simulink model "Test_Linear_system"  (R2022b)
settings: Solver=VariableStepAuto  StartTime=0.0  StopTime=50  RelTol=1e-3
values from neighbouring files (symbols this model uses):
  A = double(A)    [sys_Modelling.m]
  B = double(B)    [sys_Modelling.m]
  C = zeros((N+1)*n, N*p)    [MPC_Matrices.m]    (also in sys_Modelling.m = double(C))
  D = double(D)    [sys_Modelling.m]
  L = place(sys.A', sys.C',ew_L)'    [Controller_Observer.m]    (also in LQR_Luenberger.m)
  V = -pinv(sys.C*inv(sys.A - sys.B*K)*sys.B)    [Controller_Observer.m]    (also in LQR_Luenberger.m)
undefined symbols (not defined in the file or in its folder): K_neu, u_ap
libraries: simulink_extras x2
settings Model: Creator=renzhijian  LastModifiedBy=12056

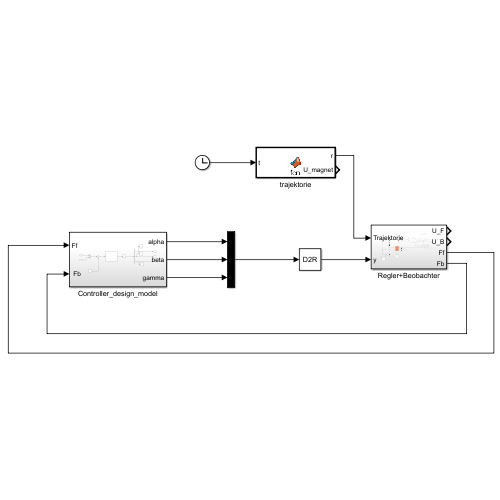
[thumbnail: Simulink's stored preview of the top-level diagram]
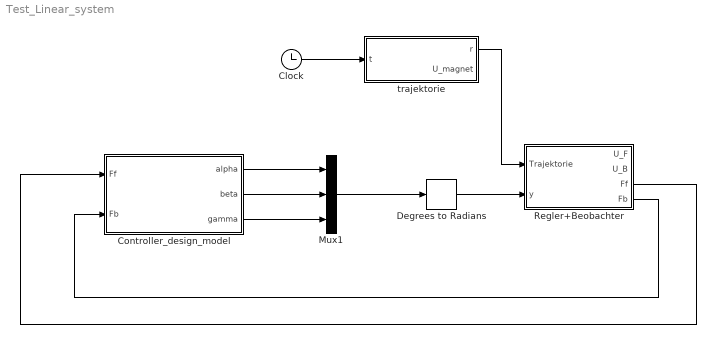
== system Test_Linear_system ==
  Clock : Clock
  Controller_design_model : Subsystem
  Degrees to Radians : simulink_extras/Transformations/Degrees to Radians
  Mux1 : Mux  Inputs=3
  Regler+Beobachter : Subsystem
  trajektorie : MATLAB Function  TreatAsAtomicUnit=on
  wires:
  Controller_design_model/1(alpha) -> Mux1/1
  trajektorie/1(r) -> Regler+Beobachter/1(Trajektorie)
  Regler+Beobachter/3(Ff) -> Controller_design_model/1(Ff)
  Controller_design_model/2(beta) -> Mux1/2
  Controller_design_model/3(gamma) -> Mux1/3
  Regler+Beobachter/4(Fb) -> Controller_design_model/2(" Fb")
  Clock/1 -> trajektorie/1(t)
  Mux1/1 -> Degrees to Radians/1
  Degrees to Radians/1 -> Regler+Beobachter/2(y)

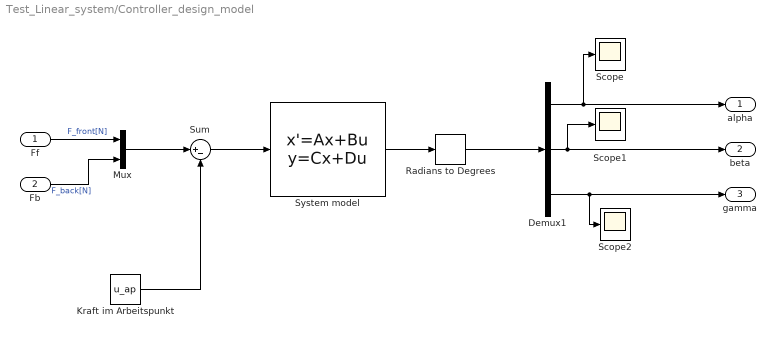
== system Test_Linear_system/Controller_design_model ==
  Ff : Inport
  " Fb" : Inport  Port=2
  Demux1 : Demux  Outputs=3
  Kraft im Arbeitspunkt : Constant  Value=u_ap
  Mux : Mux  Inputs=2
  Radians to Degrees : simulink_extras/Transformations/Radians to Degrees
  Scope : Scope
  Scope1 : Scope
  Scope2 : Scope
  Sum : Sum  Inputs=|+-
  System model : StateSpace  A=A  B=B  C=C  D=D  InitialCondition=[0;-27*pi/180;0;0;0;0]
  alpha : Outport  VectorParamsAs1DForOutWhenUnconnected=off
  beta : Outport  Port=2  VectorParamsAs1DForOutWhenUnconnected=off
  gamma : Outport  Port=3  VectorParamsAs1DForOutWhenUnconnected=off
  wires:
  " Fb"/1 -> Mux/2  "F_back[N]"
  Kraft im Arbeitspunkt/1 -> Sum/2
  System model/1 -> Radians to Degrees/1
  Sum/1 -> System model/1
  Mux/1 -> Sum/1
  Demux1/2 -> beta/1, Scope1/1
  Demux1/3 -> Scope2/1, gamma/1
  Ff/1 -> Mux/1  "F_front[N]"
  Demux1/1 -> Scope/1, alpha/1
  Radians to Degrees/1 -> Demux1/1

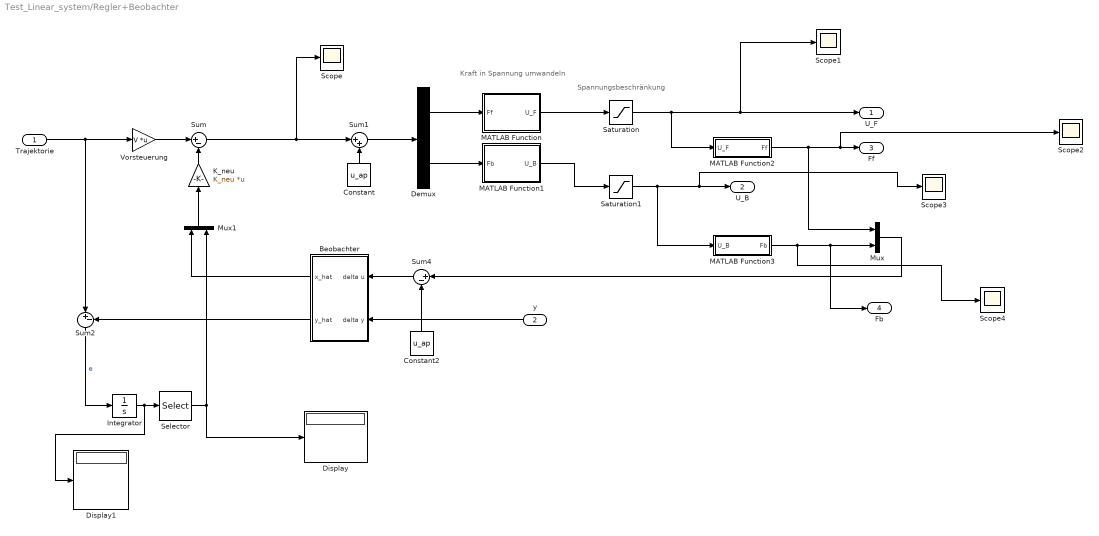
== system Test_Linear_system/Regler+Beobachter ==
  note: Spannungsbeschränkung
  note: Kraft in Spannung umwandeln
  Trajektorie : Inport
  y : Inport  Port=2
  Beobachter : Subsystem
  Constant : Constant  Value=u_ap
  Constant2 : Constant  Value=u_ap
  Demux : Demux  Outputs=2
  Display : Display
  Display1 : Display
  Integrator : Integrator
  K_neu : Gain  Gain=K_neu  Multiplication=Matrix(K*u) (u vector)
  MATLAB Function : MATLAB Function  TreatAsAtomicUnit=on
  MATLAB Function1 : MATLAB Function  TreatAsAtomicUnit=on
  MATLAB Function2 : MATLAB Function  TreatAsAtomicUnit=on
  MATLAB Function3 : MATLAB Function  TreatAsAtomicUnit=on
  Mux : Mux  Inputs=2
  Mux1 : Mux  Inputs=2
  Saturation : Saturate  UpperLimit=4  LowerLimit=0
  Saturation1 : Saturate  UpperLimit=4  LowerLimit=0
  Scope{,1..4} (5 alike) : Scope
  Selector : Selector  InputPortWidth=3  IndexOptions=Index vector (dialog)  Indices=[1 2]  OutputSizes=1
  Sum : Sum  Inputs=|+-
  Sum1 : Sum  Inputs=|++
  Sum2 : Sum  Inputs=|+-
  Sum4 : Sum  Inputs=|+-
  Vorsteuerung : Gain  Gain=V  Multiplication=Matrix(K*u) (u vector)
  U_F : Outport
  U_B : Outport  Port=2
  Ff : Outport  Port=3
  Fb : Outport  Port=4
  wires:
  MATLAB Function1/1(U_B) -> Saturation1/1
  y/1 -> Beobachter/2(delta y)
  Saturation1/1 -> MATLAB Function3/1(U_B), Scope3/1, U_B/1
  Demux/1 -> MATLAB Function/1(Ff)
  Sum1/1 -> Demux/1
  Saturation/1 -> Scope1/1, U_F/1, MATLAB Function2/1(U_F)
  Mux/1 -> Sum4/1
  MATLAB Function2/1(Ff) -> Scope2/1, Ff/1, Mux/1
  MATLAB Function3/1(Fb) -> Scope4/1, Fb/1, Mux/2
  Constant2/1 -> Sum4/2
  Constant/1 -> Sum1/2
  MATLAB Function/1(U_F) -> Saturation/1
  Sum4/1 -> Beobachter/1(delta u)
  Demux/2 -> MATLAB Function1/1(Fb)
  Trajektorie/1 -> Vorsteuerung/1, Sum2/1
  Sum/1 -> Scope/1, Sum1/1
  Sum2/1 -> Integrator/1  "e"
  Integrator/1 -> Display1/1, Selector/1
  Beobachter/2(y_hat) -> Sum2/2
  Beobachter/1(x_hat) -> Mux1/1
  Mux1/1 -> K_neu/1
  K_neu/1 -> Sum/2
  Vorsteuerung/1 -> Sum/1
  Selector/1 -> Mux1/2, Display/1

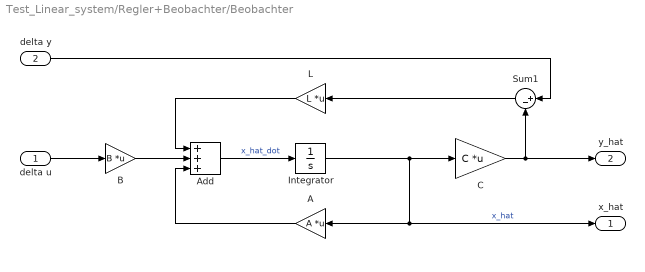
== system Test_Linear_system/Regler+Beobachter/Beobachter ==
  delta u : Inport
  delta y : Inport  Port=2
  A : Gain  Gain=A  Multiplication=Matrix(K*u) (u vector)
  Add : Sum  Inputs=+++
  B : Gain  Gain=B  Multiplication=Matrix(K*u) (u vector)
  C : Gain  Gain=C  Multiplication=Matrix(K*u) (u vector)
  Integrator : Integrator  InitialCondition=[0;-27*pi/180;0;0;0;0]
  L : Gain  Gain=L  Multiplication=Matrix(K*u) (u vector)
  Sum1 : Sum  Inputs=|+-
  x_hat : Outport
  y_hat : Outport  Port=2
  wires:
  Integrator/1 -> x_hat/1, A/1, C/1  "x_hat"
  L/1 -> Add/1
  Add/1 -> Integrator/1  "x_hat_dot"
  delta u/1 -> B/1
  Sum1/1 -> L/1
  A/1 -> Add/3
  B/1 -> Add/2
  delta y/1 -> Sum1/1
  C/1 -> y_hat/1, Sum1/2

== matlab function Test_Linear_system/Regler+Beobachter/MATLAB Function ==
  data: Ff input; U_F output
function U_F = fcn(Ff)
if Ff<0
    U_F= -(10000/733*abs(Ff))^(1/2);
else
    U_F= (10000/733*abs(Ff))^(1/2);
end

== matlab function Test_Linear_system/Regler+Beobachter/MATLAB Function1 ==
  data: Fb input; U_B output
function U_B = fcn(Fb)
if Fb<0
    U_B= -sqrt(1000/66*abs(Fb));
else
    U_B= sqrt(1000/66*abs(Fb));
end

== matlab function Test_Linear_system/Regler+Beobachter/MATLAB Function2 ==
  data: U_F input; Ff output
function Ff = fcn(U_F)
if U_F<0
    Ff = -0.0733*U_F^2;
else
    Ff = 0.0733*U_F^2;
end

== matlab function Test_Linear_system/Regler+Beobachter/MATLAB Function3 ==
  data: U_B input; Fb output
function Fb = fcn(U_B)
if U_B<0
    Fb = -0.066*U_B^2;
else
    Fb = 0.066*U_B^2;
end

== matlab function Test_Linear_system/trajektorie ==
  data: t input; r output; U_magnet output
function [r, U_magnet] = fcn(t)
beta = -27;
if t <= 10
    a0 = five_times_plan(0, -27, 0, 0, 10, 0, 0, 0);
    alpha = 0;
    beta = a0(1)+a0(2)*t+a0(3)*t^2+a0(4)*t^3+a0(5)*t^4+a0(6)*t^5;
    U_magnet = 0;
elseif t > 10 && t <= 18
    a0 = five_times_plan(10, 0, 0, 0, 18, 90, 0, 0);
    alpha = a0(1)+a0(2)*t+a0(3)*t^2+a0(4)*t^3+a0(5)*t^4+a0(6)*t^5;
    beta = 0;
    U_magnet = 0;
elseif t > 18 &&t <= 26
    a0 = five_times_plan(18, 0, 0, 0, 26, -22, 0, 0);
    alpha = 90;
    beta = a0(1)+a0(2)*t+a0(3)*t^2+a0(4)*t^3+a0(5)*t^4+a0(6)*t^5;
    U_magnet = 1;
elseif t > 26 && t <= 30
    alpha = 90;
    beta = -22;
    U_magnet = 0;
elseif t > 30 && t <= 38
    a0 = five_times_plan(30, -22, 0, 0, 38, 0, 0, 0);
    alpha = 90;
    beta = a0(1)+a0(2)*t+a0(3)*t^2+a0(4)*t^3+a0(5)*t^4+a0(6)*t^5;
    U_magnet = 0;
elseif t > 38 && t <= 62
    a0 = five_times_plan(38, 90, 0, 0,62, 450, 0, 0);
    alpha = a0(1)+a0(2)*t+a0(3)*t^2+a0(4)*t^3+a0(5)*t^4+a0(6)*t^5;
    beta = 0;
    U_magnet = 0;
elseif t > 62 && t <= 70
    a0 = five_times_plan(62, 0, 0, 0, 70, -22, 0, 0); 
    alpha = 450;
    beta = a0(1)+a0(2)*t+a0(3)*t^2+a0(4)*t^3+a0(5)*t^4+a0(6)*t^5;
    U_magnet = 1;
elseif t > 70 && t <= 74
    alpha = 450;
    beta = -22;
    U_magnet = 0;
elseif t > 74 && t <= 82
    a0 = five_times_plan(74, -22, 0, 0, 82, 0, 0, 0);
    alpha = 450;
    beta = a0(1)+a0(2)*t+a0(3)*t^2+a0(4)*t^3+a0(5)*t^4+a0(6)*t^5;
    U_magnet = 0;
elseif t > 82 && t <= 110
    a0 = five_times_plan(82, 450, 0, 0, 110, 0, 0, 0);
    alpha = a0(1)+a0(2)*t+a0(3)*t^2+a0(4)*t^3+a0(5)*t^4+a0(6)*t^5;
    beta = 0;
    U_magnet = 0;
elseif t > 110 && t < 118
    a0 = five_times_plan(110, 0, 0, 0, 118, -27, 0, 0);
    alpha = 0;
    beta = a0(1)+a0(2)*t+a0(3)*t^2+a0(4)*t^3+a0(5)*t^4+a0(6)*t^5;
    U_magnet = 1;
else 
    alpha = 0; beta = -27;
    U_magnet = 0;
end
r = [alpha; beta;0];
function a = five_times_plan(ts, xs, vs, as, te, xe, ve, ae)
    para = [xs;vs;as;xe;ve;ae];
    Tran = [1,   ts,  ts^2,  ts^3,    ts^4,     ts^5;
            0,   1,   2*ts,  3*ts^2,  4*ts^3,   5*ts^4;
            0,   0,   2,     6*ts,    12*ts^2,  20*ts^3;
            1,   te,  te^2,  te^3,    te^4,     te^5;
            0,   1,   2*te,  3*te^2,  4*te^3,   5*te^4;
            0,   0,   2,     6*te,    12*te^2,  20*te^3];
    a = inv(Tran)*para;
end
end
